simulink model "tracking_model"  (R2017a)
settings: Solver=VariableStepAuto  StartTime=0.0  StopTime=10.0  RelTol=1e-3
undefined symbols (not defined in the file or in its folder): sys, x0
(part 2 of 14)

== matlab function tracking_model/control_function ==
  data: in1 input; u output; in2 input

function u = ControlFunction(in1,in2)

%    This function was generated by the Symbolic Math Toolbox version 7.2.

%    10-Jan-2021 16:43:15



th_ref = in2(3,:);

thp_ref = in2(6,:);

thpp_ref = in2(9,:);

x_1 = in1(1,:);

x_2 = in1(2,:);

x_3 = in1(3,:);

x_4 = in1(4,:);

x_5 = in1(5,:);

x_6 = in1(6,:);

x_7 = in1(7,:);

x_8 = in1(8,:);

x_9 = in1(9,:);

x_ref = in2(1,:);

xp_ref = in2(4,:);

xpp_ref = in2(7,:);

y_ref = in2(2,:);

yp_ref = in2(5,:);

ypp_ref = in2(8,:);

